simulink model "PROVA_SORPASSO_V2"  (R2019b)
settings: Solver=ode4  StartTime=0.0  StopTime=T  FixedStep=Tc  RelTol=1e-3
values from neighbouring files (symbols this model uses):
  acc_A = acc_A_all(i)    [TEST_AUTOMATICO.m]
  acc_B = acc_B_all(i)    [TEST_AUTOMATICO.m]
  init_sim = [X0 (V0_ego_init/3.6) Angles0]'    [TEST_AUTOMATICO.m]
  init_sim_A = [X0_A (V0_A_init/3.6) Angles0_A]'    [TEST_AUTOMATICO.m]
  init_sim_B = [X0_B (V0_B_init/3.6) Angles0_B]'    [TEST_AUTOMATICO.m]
  T = 30    [TEST_AUTOMATICO.m]
  Tc = 0.1    [TEST_AUTOMATICO.m]
  V0_A_init = V0_A(i)    [TEST_AUTOMATICO.m]
  V0_B_init = V0_B(i)    [TEST_AUTOMATICO.m]
  V0_ego_init = V0_ego(i)    [TEST_AUTOMATICO.m]
  xx_rif = 0 : Tc : x_tr(end)    [TEST_AUTOMATICO.m]
  xx_rif_A = 0:Tc:(x_tr_A(end))    [TEST_AUTOMATICO.m]
  xx_rif_B = 1000:-Tc:0    [TEST_AUTOMATICO.m]
  yy_rif_B = ones(size(xx_rif_B,1),size(xx_rif_B,2))*6    [TEST_AUTOMATICO.m]
undefined symbols (not defined in the file or in its folder): yy_rif, yy_rif_A
libraries: simulink x2, mpcadaslib x1
settings Model: Creator=The MathWorks, Inc.  LastModifiedBy=mario
settings DataIOCC: ReturnWorkspaceOutputs=off
settings DebuggingCC: ArithmeticOperatorsInVariantConditions=warning
settings SFSimCC: SimUseLocalCustomCode=off  CustomCodeUndefinedFunction=UseInterfaceOnly
settings RTWCC: RTWUseLocalCustomCode=off
settings CodeAppCC: StateflowObjectComments=on

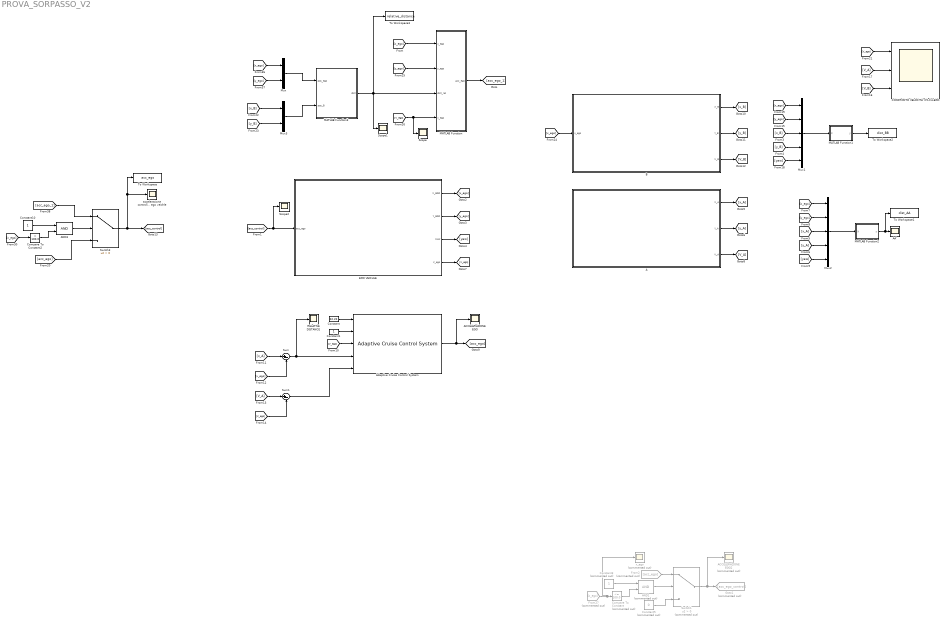
== system PROVA_SORPASSO_V2 ==
  A : Subsystem
  AA' : Scope
  ACCELERAZIONE EGO : Scope
  ACCELERAZIONE EGO2 : Scope  Commented=on
  AND1 : Logic  Commented=on  IconShape=distinctive  AllPortsSameDT=off  OutDataTypeStr=boolean
  AND3 : Logic  IconShape=distinctive  AllPortsSameDT=off  OutDataTypeStr=boolean
  Adaptive Cruise Control System : mpcadaslib/Adaptive Cruise Control System  EgoModel=tf(1,[0.5,1,0])  InitialEgoVelocity=(V0_ego_init/3.6)  DefaultSpacing=3  MaxVelocity=22.22  MinAcceleration=-4  amin_ext=off  MaxAcceleration=2  amax_ext=off  Ts=Tc  PredictionHorizon=60  ControllerBehavior=0.180  suboptimal=off  maxiter=10  datatypeopt=double  optmode=off  trackmode=off
      settings: SourceProductName=Model Predictive Control Toolbox
  B : Subsystem
  CONFRONTO VELOCITA' C5-C4-EGO : Scope  NumInputPorts=3
  Compare To Constant : simulink/Logic and Bit Operations/Compare To Constant  Commented=on  relop=<=  const=100.0  OutDataTypeStr=boolean
  Compare To Constant2 : simulink/Logic and Bit Operations/Compare To Constant  relop=>  const=100.0  OutDataTypeStr=boolean
  Constant : Constant  Value=22.22
  Constant1 : Constant
  Constant10 : Constant
  Constant3 : Constant  Commented=on
  Constant5 : Constant  Commented=on  Value=0
  EGO VEICHLE : Subsystem
  From2 : From  Commented=on  GotoTag=acc_ego
  From27 : From  Commented=on  GotoTag=x_ego
  Goto1 : Goto  Commented=on  GotoTag=acc_ego_control
  MATLAB Function : MATLAB Function  TreatAsAtomicUnit=on
  MATLAB Function1 : MATLAB Function  TreatAsAtomicUnit=on
  MATLAB Function2 : MATLAB Function  TreatAsAtomicUnit=on
  MATLAB Function3 : MATLAB Function  TreatAsAtomicUnit=on
  Mux : Mux  Inputs=2
  Mux1 : Mux  Inputs=5
  Mux2 : Mux  Inputs=5
  Mux3 : Mux  Inputs=2
  RELATIVE DISTANCE : Scope
  Scope : Scope
  Scope1 : Scope
  Scope2 : Scope
  Sum : Sum  Inputs=|+-
  Sum1 : Sum  Inputs=|+-
  Switch1 : Switch  Commented=on  Criteria=u2 > Threshold
  Switch3 : Switch  Criteria=u2 > Threshold
  To Workspace : ToWorkspace  VariableName=acc_ego  SaveFormat=Structure With Time  SampleTime=Tc
  To Workspace1 : ToWorkspace  VariableName=dist_AA  SaveFormat=Structure With Time  SampleTime=-1
  To Workspace2 : ToWorkspace  VariableName=dist_BB  SaveFormat=Structure With Time  SampleTime=-1
  To Workspace3 : ToWorkspace  VariableName=relative_distance  SaveFormat=Structure With Time  SampleTime=-1
  accelerazione controllo ego veichle : Scope
  x_ego : Scope  Commented=on
  wires:
  EGO VEICHLE/1(X_EGO) -> [x_ego]
  EGO VEICHLE/2(Y_EGO) -> [y_ego]
  EGO VEICHLE/3(YAW) -> [yaw]
  A/1(X_A) -> [x_A]
  A/2("Y_A ") -> [y_A]
  [x_A] -> Mux2/3
  Mux2/1 -> MATLAB Function2/1(X)
  MATLAB Function2/1(y) -> To Workspace1/1, AA'/1
  [y_ego] -> Mux2/2
  [yaw] -> Mux2/5
  [x_ego] -> Mux2/1
  [y_A] -> Mux2/4
  Constant/1 -> Adaptive Cruise Control System/1
  Constant1/1 -> Adaptive Cruise Control System/2
  EGO VEICHLE/4(V_ego) -> [V_ego]
  [V_ego] -> Adaptive Cruise Control System/3
  [x_ego] -> Sum/2
  Sum/1 -> RELATIVE DISTANCE/1, Adaptive Cruise Control System/4
  A/3(V_A) -> [V_A]
  [V_A] -> Sum1/1
  [V_ego] -> Sum1/2
  Sum1/1 -> Adaptive Cruise Control System/5
  Adaptive Cruise Control System/1 -> [acc_ego], ACCELERAZIONE EGO/1
  AND1/1 -> Switch1/2
  Switch1/1 -> Goto1/1, ACCELERAZIONE EGO2/1
  From27/1 -> x_ego/1, Compare To Constant/1
  Constant5/1 -> Switch1/3
  From2/1 -> Switch1/1
  Constant3/1 -> AND1/1
  Compare To Constant/1 -> AND1/2
  [yaw] -> Mux1/5
  Mux1/1 -> MATLAB Function1/1(X)
  MATLAB Function1/1(y) -> To Workspace2/1
  [y_ego] -> Mux1/2
  B/2("Y_B ") -> [y_B]
  B/1("X_B ") -> [x_B]
  B/3(V_B) -> [V_B]
  [x_B] -> Mux1/3
  [x_ego] -> Mux1/1
  AND3/1 -> Switch3/2
  Compare To Constant2/1 -> AND3/2
  [x_ego] -> Compare To Constant2/1
  Constant10/1 -> AND3/1
  Switch3/1 -> [acc_control], accelerazione controllo ego veichle/1, To Workspace/1
  [x_ego] -> MATLAB Function/1(x_ego)
  [y_ego] -> MATLAB Function/2(y_ego)
  [V_ego] -> Scope/1, MATLAB Function/4(v_ego)
  MATLAB Function/1(acc_ego) -> [acc_ego_1]
  [acc_ego_1] -> Switch3/1
  [acc_ego] -> Switch3/3
  [y_ego] -> Mux/2
  [x_ego] -> Mux/1
  Mux/1 -> MATLAB Function3/1(pos_ego)
  Mux3/1 -> MATLAB Function3/2(pos_B)
  MATLAB Function3/1(dist) -> To Workspace3/1, Scope1/1, MATLAB Function/3(dist_rel)
  [y_B] -> Mux1/4
  [acc_control] -> Scope2/1, EGO VEICHLE/1(acc_ego)
  [V_B] -> CONFRONTO VELOCITA' C5-C4-EGO/3
  [V_A] -> CONFRONTO VELOCITA' C5-C4-EGO/2
  [V_ego] -> CONFRONTO VELOCITA' C5-C4-EGO/1
  [x_A] -> Sum/1
  [y_B] -> Mux3/2
  [x_B] -> Mux3/1
  [x_ego] -> B/1(x_ego)

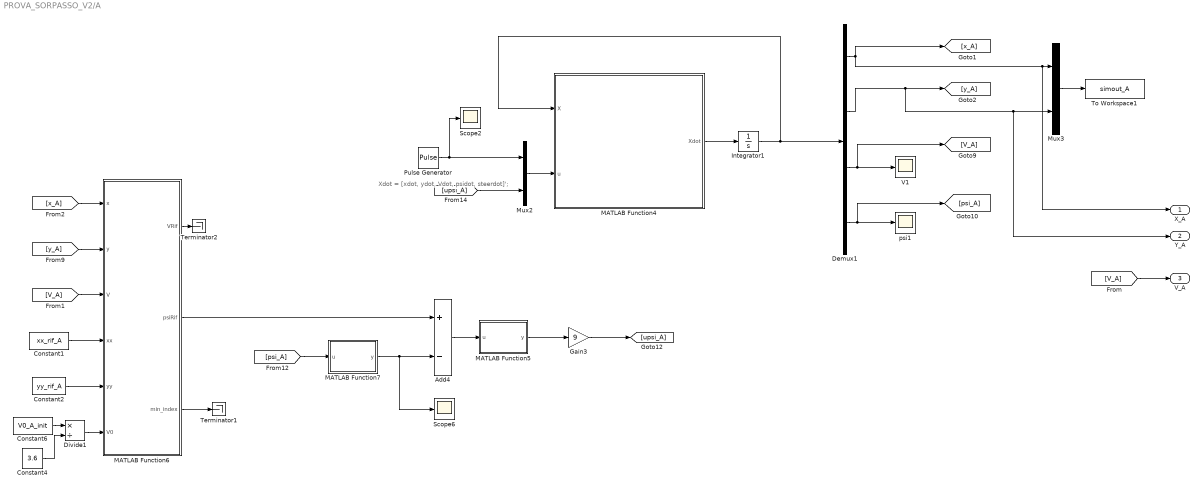
== system PROVA_SORPASSO_V2/A ==
  note: Xdot = [xdot, ydot, Vdot, psidot, steerdot]';
  Add4 : Sum  Inputs=+-
  Constant1 : Constant  Value=xx_rif_A
  Constant2 : Constant  Value=yy_rif_A
  Constant4 : Constant  Value=3.6
  Constant6 : Constant  Value=V0_A_init
  Demux1 : Demux
  Divide1 : Product  Inputs=*/
  Gain3 : Gain  Gain=9
  Integrator1 : Integrator  InitialCondition=init_sim_A
  MATLAB Function4 : MATLAB Function  TreatAsAtomicUnit=on
  MATLAB Function5 : MATLAB Function  TreatAsAtomicUnit=on
  MATLAB Function6 : MATLAB Function  TreatAsAtomicUnit=on
  MATLAB Function7 : MATLAB Function  TreatAsAtomicUnit=on
  Mux2 : Mux  Inputs=2
  Mux3 : Mux  Inputs=2
  Pulse Generator : DiscretePulseGenerator  PulseType=Time based  Amplitude=acc_A  Period=T  PulseWidth=3
  Scope2 : Scope
  Scope6 : Scope
  Terminator1 : Terminator
  Terminator2 : Terminator
  To Workspace1 : ToWorkspace  VariableName=simout_A  SaveFormat=Structure With Time  SampleTime=-1
  V1 : Scope
  psi1 : Scope
  X_A : Outport
  "Y_A " : Outport  Port=2
  V_A : Outport  Port=3
  wires:
  [upsi_A] -> Mux2/2
  [psi_A] -> MATLAB Function7/1(u)
  MATLAB Function7/1(y) -> Scope6/1, Add4/2
  MATLAB Function6/3(min_index) -> Terminator1/1
  Mux3/1 -> To Workspace1/1
  [x_A] -> MATLAB Function6/1(x)
  Demux1/3 -> V1/1, [V_A]
  MATLAB Function4/1(Xdot) -> Integrator1/1
  [V_A] -> MATLAB Function6/3(V)
  Demux1/4 -> [psi_A], psi1/1
  Demux1/1 -> X_A/1, Mux3/1, [x_A]
  Mux2/1 -> MATLAB Function4/2(u)
  Demux1/2 -> [y_A], "Y_A "/1, Mux3/2
  [y_A] -> MATLAB Function6/2(y)
  Integrator1/1 -> Demux1/1, MATLAB Function4/1(X)
  Add4/1 -> MATLAB Function5/1(u)
  Gain3/1 -> [upsi_A]
  Constant1/1 -> MATLAB Function6/4(xx)
  MATLAB Function6/2(psiRif) -> Add4/1
  Constant2/1 -> MATLAB Function6/5(yy)
  MATLAB Function5/1(y) -> Gain3/1
  [V_A] -> V_A/1
  Pulse Generator/1 -> Mux2/1, Scope2/1
  Constant4/1 -> Divide1/2
  Constant6/1 -> Divide1/1
  Divide1/1 -> MATLAB Function6/6(V0)
  MATLAB Function6/1(VRif) -> Terminator2/1

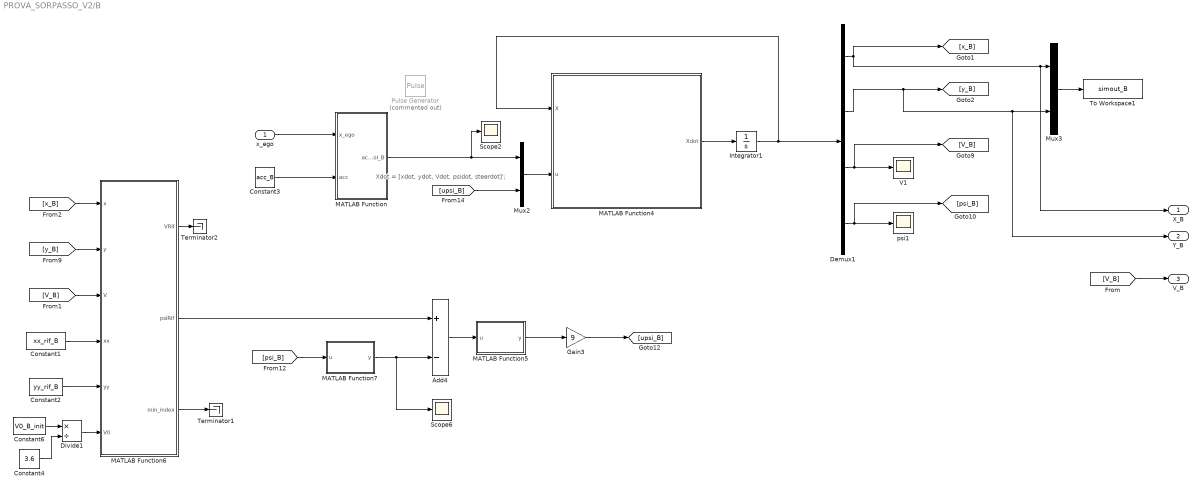
== system PROVA_SORPASSO_V2/B ==
  note: Xdot = [xdot, ydot, Vdot, psidot, steerdot]';
  x_ego : Inport
  Add4 : Sum  Inputs=+-
  Constant1 : Constant  Value=xx_rif_B
  Constant2 : Constant  Value=yy_rif_B
  Constant3 : Constant  Value=acc_B
  Constant4 : Constant  Value=3.6
  Constant6 : Constant  Value=V0_B_init
  Demux1 : Demux
  Divide1 : Product  Inputs=*/
  Gain3 : Gain  Gain=9
  Integrator1 : Integrator  InitialCondition=init_sim_B
  MATLAB Function : MATLAB Function  TreatAsAtomicUnit=on
  MATLAB Function4 : MATLAB Function  TreatAsAtomicUnit=on
  MATLAB Function5 : MATLAB Function  TreatAsAtomicUnit=on
  MATLAB Function6 : MATLAB Function  TreatAsAtomicUnit=on
  MATLAB Function7 : MATLAB Function  TreatAsAtomicUnit=on
  Mux2 : Mux  Inputs=2
  Mux3 : Mux  Inputs=2
  Pulse Generator : DiscretePulseGenerator  Commented=on  PulseType=Time based  Amplitude=acc_B  Period=T  PulseWidth=2  PhaseDelay=6
  Scope2 : Scope
  Scope6 : Scope
  Terminator1 : Terminator
  Terminator2 : Terminator
  To Workspace1 : ToWorkspace  VariableName=simout_B  SaveFormat=Structure With Time  SampleTime=-1
  V1 : Scope
  psi1 : Scope
  "X_B " : Outport
  "Y_B " : Outport  Port=2
  V_B : Outport  Port=3
  wires:
  [upsi_B] -> Mux2/2
  [psi_B] -> MATLAB Function7/1(u)
  MATLAB Function7/1(y) -> Scope6/1, Add4/2
  MATLAB Function6/3(min_index) -> Terminator1/1
  Mux3/1 -> To Workspace1/1
  [x_B] -> MATLAB Function6/1(x)
  Demux1/3 -> V1/1, [V_B]
  MATLAB Function4/1(Xdot) -> Integrator1/1
  [V_B] -> MATLAB Function6/3(V)
  Demux1/4 -> [psi_B], psi1/1
  Demux1/1 -> "X_B "/1, Mux3/1, [x_B]
  Mux2/1 -> MATLAB Function4/2(u)
  Demux1/2 -> [y_B], "Y_B "/1, Mux3/2
  [y_B] -> MATLAB Function6/2(y)
  Integrator1/1 -> Demux1/1, MATLAB Function4/1(X)
  Add4/1 -> MATLAB Function5/1(u)
  Gain3/1 -> [upsi_B]
  Constant1/1 -> MATLAB Function6/4(xx)
  MATLAB Function6/2(psiRif) -> Add4/1
  Constant2/1 -> MATLAB Function6/5(yy)
  MATLAB Function5/1(y) -> Gain3/1
  [V_B] -> V_B/1
  Constant4/1 -> Divide1/2
  Constant6/1 -> Divide1/1
  Divide1/1 -> MATLAB Function6/6(V0)
  MATLAB Function6/1(VRif) -> Terminator2/1
  x_ego/1 -> MATLAB Function/1(x_ego)
  Constant3/1 -> MATLAB Function/2(acc)
  MATLAB Function/1(acc_control_B) -> Scope2/1, Mux2/1

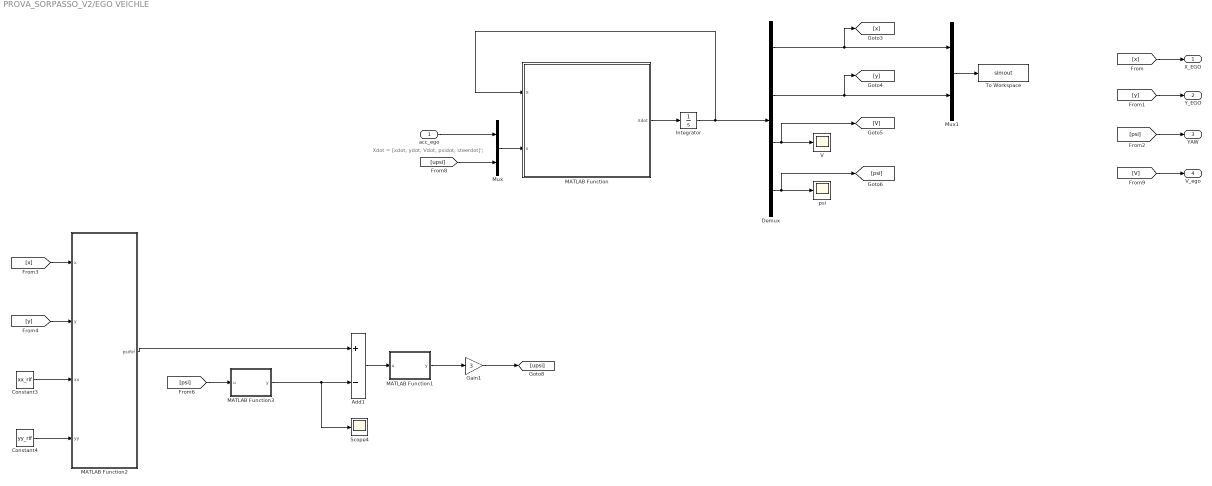
== system PROVA_SORPASSO_V2/EGO VEICHLE ==
  note: Xdot = [xdot, ydot, Vdot, psidot, steerdot]';
  acc_ego : Inport
  Add1 : Sum  Inputs=+-
  Constant3 : Constant  Value=xx_rif
  Constant4 : Constant  Value=yy_rif
  Demux : Demux
  Gain1 : Gain  Gain=3
  Integrator : Integrator  InitialCondition=init_sim
  MATLAB Function : MATLAB Function  TreatAsAtomicUnit=on
  MATLAB Function1 : MATLAB Function  TreatAsAtomicUnit=on
  MATLAB Function2 : MATLAB Function  TreatAsAtomicUnit=on
  MATLAB Function3 : MATLAB Function  TreatAsAtomicUnit=on
  Mux : Mux  Inputs=2
  Mux1 : Mux  Inputs=2
  Scope4 : Scope
  To Workspace : ToWorkspace  VariableName=simout  SaveFormat=Structure With Time  SampleTime=-1
  V : Scope
  psi : Scope
  X_EGO : Outport
  Y_EGO : Outport  Port=2
  YAW : Outport  Port=3
  V_ego : Outport  Port=4
  wires:
  Constant4/1 -> MATLAB Function2/4(yy)
  Demux/1 -> Mux1/1, [x]
  [upsi] -> Mux/2
  MATLAB Function3/1(y) -> Scope4/1, Add1/2
  Integrator/1 -> Demux/1, MATLAB Function/1(X)
  Gain1/1 -> [upsi]
  Demux/4 -> [psi], psi/1
  Constant3/1 -> MATLAB Function2/3(xx)
  Demux/2 -> [y], Mux1/2
  Demux/3 -> V/1, [V]
  [y] -> MATLAB Function2/2(y)
  Mux/1 -> MATLAB Function/2(u)
  MATLAB Function/1(Xdot) -> Integrator/1
  acc_ego/1 -> Mux/1
  [x] -> MATLAB Function2/1(x)
  Mux1/1 -> To Workspace/1
  MATLAB Function1/1(y) -> Gain1/1
  MATLAB Function2/1(psiRif) -> Add1/1
  [psi] -> MATLAB Function3/1(u)
  Add1/1 -> MATLAB Function1/1(u)
  [x] -> X_EGO/1
  [y] -> Y_EGO/1
  [psi] -> YAW/1
  [V] -> V_ego/1

== matlab function PROVA_SORPASSO_V2/EGO VEICHLE/MATLAB Function1 ==
  data: u input; y output
function y = wrapPi(u)
y = wrap_Pi(u);
end

== matlab function PROVA_SORPASSO_V2/EGO VEICHLE/MATLAB Function ==
  data: X input; u input; Xdot output
function Xdot = fcn(X,u)

L = 2.5;                     %%% lunghezza del veicolo

x = X(1);
y = X(2);
V = X(3);
psi = X(4);                  %%% angolo di imbardata
% steer = X(5);

xdot = V*cos(psi);
ydot = V*sin(psi);
Vdot = u(1);                 %%% non ci sono variazioni del modulo della velocità
psidot = u(2);

% psidot = (V/L)*tan(steer);  
% steerdot = u(2);

% Xdot = [xdot, ydot, Vdot, psidot, steerdot]';   
Xdot = [xdot, ydot, Vdot, psidot]';

end

== matlab function PROVA_SORPASSO_V2/EGO VEICHLE/MATLAB Function2 ==
  data: x input; y input; xx input; yy input; psiRif output
function psiRif  = pathfollower_mono(x, y,  xx, yy)

n = length(xx);
d_ref = zeros(1,n);

for i = 1:n
d_ref(i)= sqrt((xx(i)-x)^2+(yy(i)-y)^2);
end

[~, min_index] = min(d_ref);

min_index = min(min_index + 1, n);                                                        %%% per dargli una curva più smooth gli do qualche punto più avanti invece di quello attuale
psiRif = wrap_2Pi(atan2((yy(min_index)-y),(xx(min_index)-x)));


end






% m = length(V0)
% for j = 1:m
%    if d_ref(end)<0.1     %%% errore di riferimento
%      VRif=0;
%    else
%     VRif=V0(j);
%    end
% end
% 
% 
% % if d_ref(end)<0.1     %%% errore di riferimento
% % VRif=0;
% % else
% % VRif=V0;
% % end

== matlab function PROVA_SORPASSO_V2/B/MATLAB Function4 ==
  data: X input; u input; Xdot output
function Xdot = fcn(X,u)

L = 2.5;

x = X(1);
y = X(2);
V = X(3);
psi = X(4);                  %%% imbardata
% steer = X(5);

xdot = V*cos(psi);
ydot = V*sin(psi);
Vdot = u(1);                 %%% non ci sono variazioni del modulo della velocità
psidot = u(2);

% psidot = (V/L)*tan(steer);  
% steerdot = u(2);

% Xdot = [xdot, ydot, Vdot, psidot, steerdot]';
Xdot = [xdot, ydot, Vdot, psidot]';

end

== matlab function PROVA_SORPASSO_V2/EGO VEICHLE/MATLAB Function3 ==
  data: u input; y output
function y = wrap2Pi(u)
y = wrap_2Pi(u);
end

== matlab function PROVA_SORPASSO_V2/B/MATLAB Function5 ==
  data: u input; y output
function y = wrapPi(u)
y = wrap_Pi(u);
end

== matlab function PROVA_SORPASSO_V2/B/MATLAB Function6 ==
  data: x input; VRif output; y input; V input; xx input; yy input; V0 input; psiRif output; min_index output
function [VRif,psiRif,min_index] = pathfollower_mono(x, y, V, xx, yy,V0)

n = length(xx);
d_ref = zeros(1,n);

for i = 1:n
d_ref(i)= sqrt((xx(i)-x)^2+(yy(i)-y)^2);
end

[~, min_index] = min(d_ref);

m = length(V0)
for j = 1:m
   if d_ref(end)<0.1     %%% errore di riferimento
     VRif=0;
   else
    VRif=V0(j);
   end
end


% if d_ref(end)<0.1     %%% errore di riferimento
% VRif=0;
% else
% VRif=V0;
% end

min_index = min(min_index + 1, n);                                  %%% per dargli una curva più smooth gli do qualche punto più avanti invece di quello attuale
psiRif = wrap_2Pi(atan2((yy(min_index)-y),(xx(min_index)-x)));

end

== matlab function PROVA_SORPASSO_V2/B/MATLAB Function7 ==
  data: u input; y output
function y = wrap2Pi(u)
y = wrap_2Pi(u);
end

== matlab function PROVA_SORPASSO_V2/MATLAB Function1 ==
  data: X input; y output
function y = fcn(X)

w_ego = 1.8 ; % larghezza auto ego
w_B = 1.8 ; % larghezza auto C7

a = 2 ; % semi-lunghezza ego
b = 2 ; % semi-lunghezza C7

x0 = X(1) ;
y0 = X(2) ;

x_B = X(3) ;
y_B = X(4) ;

theta = X(5) ;

u = sqrt(  (x0 + a*cos(theta) - (1/2)*w_ego*sin(theta) - x_B + b )^2  + ...
           (y0 + a*sin(theta) + (1/2)*w_ego*cos(theta) - y_B + (1/2)*w_B)^2   )

y = u;

== matlab function PROVA_SORPASSO_V2/A/MATLAB Function4 ==
  data: X input; u input; Xdot output
function Xdot = fcn(X,u)

L = 2.5;

x = X(1);
y = X(2);
V = X(3);
psi = X(4);                  %%% imbardata
% steer = X(5);

xdot = V*cos(psi);
ydot = V*sin(psi);
Vdot = u(1);                 %%% non ci sono variazioni del modulo della velocità
psidot = u(2);

% psidot = (V/L)*tan(steer);  
% steerdot = u(2);

% Xdot = [xdot, ydot, Vdot, psidot, steerdot]';
Xdot = [xdot, ydot, Vdot, psidot]';

end

== matlab function PROVA_SORPASSO_V2/A/MATLAB Function5 ==
  data: u input; y output
function y = wrapPi(u)
y = wrap_Pi(u);
end

== matlab function PROVA_SORPASSO_V2/A/MATLAB Function6 ==
  data: x input; VRif output; y input; V input; xx input; yy input; V0 input; psiRif output; min_index output
function [VRif,psiRif,min_index] = pathfollower_mono(x, y, V, xx, yy,V0)

n = length(xx);
d_ref = zeros(1,n);

for i = 1:n
d_ref(i)= sqrt((xx(i)-x)^2+(yy(i)-y)^2);
end

[~, min_index] = min(d_ref);

m = length(V0)
for j = 1:m
   if d_ref(end)<0.1     %%% errore di riferimento
     VRif=0;
   else
    VRif=V0(j);
   end
end


% if d_ref(end)<0.1     %%% errore di riferimento
% VRif=0;
% else
% VRif=V0;
% end

min_index = min(min_index + 1, n);                                  %%% per dargli una curva più smooth gli do qualche punto più avanti invece di quello attuale
psiRif = wrap_2Pi(atan2((yy(min_index)-y),(xx(min_index)-x)));

end

== matlab function PROVA_SORPASSO_V2/A/MATLAB Function7 ==
  data: u input; y output
function y = wrap2Pi(u)
y = wrap_2Pi(u);
end

== matlab function PROVA_SORPASSO_V2/MATLAB Function2 ==
  data: X input; y output
function y = fcn(X)

w_ego = 1.8 ; % larghezza auto ego
w_A = 1.8 ; % larghezza auto C7

a = 2 ; % semi-lunghezza ego
b = 2 ; % semi-lunghezza C7

x0 = X(1) ;
y0 = X(2) ;

x_A = X(3) ;
y_A = X(4) ;

theta = X(5) ;

u = sqrt(  (x0 + a*cos(theta) + (1/2)*w_ego*sin(theta) - x_A + b )^2  + ...
           (y0 + a*sin(theta) - (1/2)*w_ego*cos(theta) - y_A - (1/2)*w_A)^2   )

y = u;

== matlab function PROVA_SORPASSO_V2/MATLAB Function ==
  data: x_ego input; y_ego input; dist_rel input; v_ego input; acc_ego output
function acc_ego = fcn( x_ego, y_ego, dist_rel, v_ego)

acc_max = 2;

if x_ego >= 100 && x_ego <= 200 && y_ego >=2.5 && y_ego <= 6.5
    
    
    if v_ego < 33
        
        
        acc_ego =  acc_max;
        
    else
        
        acc_ego = 0;
        
    end
else
    
    acc_ego = 0;
    
end
end

== matlab function PROVA_SORPASSO_V2/MATLAB Function3 ==
  data: pos_ego input; dist output; pos_B input
function dist = fcn(pos_ego,pos_B)

    
    dist = norm(pos_ego-pos_B);


end

== matlab function PROVA_SORPASSO_V2/B/MATLAB Function ==
  data: x_ego input; acc input; acc_control_B output
function acc_control_B = fcn(x_ego, acc)

if x_ego > 100 && x_ego <= 125
    
    acc_control_B = acc;
    
else
    acc_control_B = 0;

end
